simulink model "Integrate_velocity_to_position"  (R2018a)
settings: Solver=VariableStepAuto  StartTime=0.0  StopTime=10.0  RelTol=1e-3
values from neighbouring files (symbols this model uses):
  Rearth = 6371000    [setupandrun.m]
  thetaInit_BN = thetaInit_BN_deg * deg2rad    [setupandrun.m]
  xDotInit_E_B_BE = [150; 0; 0]    [setupandrun.m]
  xInit_E_E_BE = [Rearth; 0; 0]    [setupandrun.m]
settings Model: Creator=lamy  LastModifiedBy=lamy

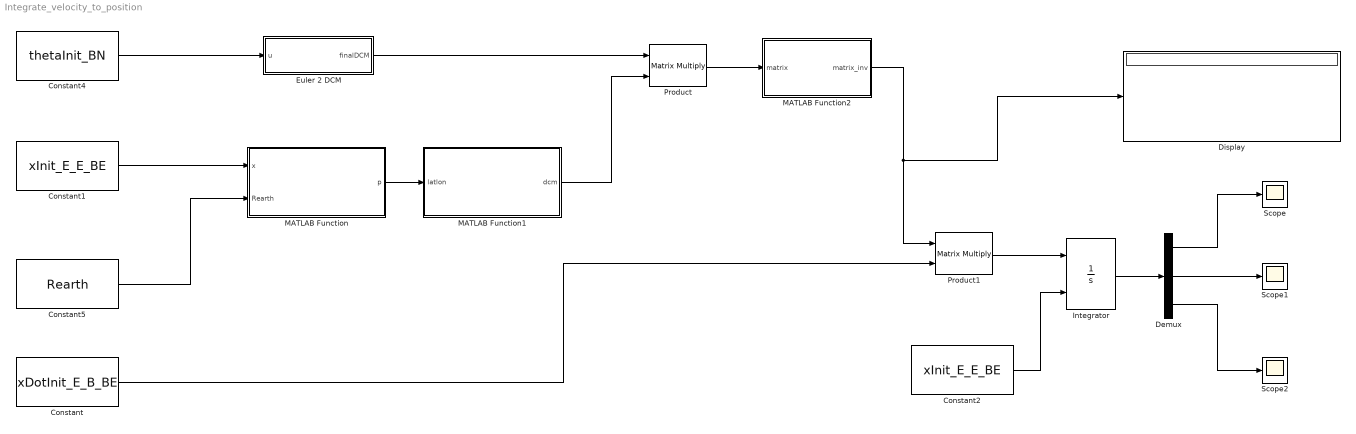
== system Integrate_velocity_to_position ==
  Constant : Constant  Value=xDotInit_E_B_BE
  Constant1 : Constant  Value=xInit_E_E_BE
  Constant2 : Constant  Value=xInit_E_E_BE
  Constant4 : Constant  Value=thetaInit_BN
  Constant5 : Constant  Value=Rearth
  Demux : Demux  Outputs=3
  Display : Display
  Euler 2 DCM : MATLAB Function  TreatAsAtomicUnit=on
  Integrator : Integrator  InitialConditionSource=external
  MATLAB Function : MATLAB Function  TreatAsAtomicUnit=on
  MATLAB Function1 : MATLAB Function  TreatAsAtomicUnit=on
  MATLAB Function2 : MATLAB Function  TreatAsAtomicUnit=on
  Product : Product  Multiplication=Matrix(*)
  Product1 : Product  Multiplication=Matrix(*)
  Scope : Scope
  Scope1 : Scope
  Scope2 : Scope
  wires:
  Constant4/1 -> Euler 2 DCM/1(u)
  Euler 2 DCM/1(finalDCM) -> Product/1
  Constant1/1 -> MATLAB Function/1(x)
  Constant5/1 -> MATLAB Function/2(Rearth)
  MATLAB Function/1(p) -> MATLAB Function1/1(latlon)
  MATLAB Function1/1(dcm) -> Product/2
  Product/1 -> MATLAB Function2/1(matrix)
  MATLAB Function2/1(matrix_inv) -> Display/1, Product1/1
  Constant/1 -> Product1/2
  Product1/1 -> Integrator/1
  Constant2/1 -> Integrator/2
  Integrator/1 -> Demux/1
  Demux/1 -> Scope/1
  Demux/2 -> Scope1/1
  Demux/3 -> Scope2/1

== matlab function Integrate_velocity_to_position/Euler 2 DCM ==
  data: u input; finalDCM output
function finalDCM = att2dcm(u)
yawDCM = [ cos(u(3)) sin(u(3)) 0 ;
-sin(u(3)) cos(u(3)) 0 ;
0 0 1 ];
pitchDCM = [ cos(u(2)) 0 -sin(u(2));
0 1 0 ;
sin(u(2)) 0 cos(u(2)) ];
rollDCM = [ 1 0 0 ;
0 cos(u(1)) sin(u(1));
0 -sin(u(1)) cos(u(1)) ];
finalDCM = rollDCM * pitchDCM * yawDCM;

== matlab function Integrate_velocity_to_position/MATLAB Function ==
  data: x input; p output; Rearth input
function p = cart2latlon(x,Rearth)
lat = atan2(x(3),sqrt(x(1)^2+x(2)^2));
lon = atan2(x(2),x(1));
alt = sqrt(x(1)^2+x(2)^2+x(3)^2) - Rearth;
p = [lat,lon,alt];

== matlab function Integrate_velocity_to_position/MATLAB Function1 ==
  data: latlon input; dcm output
function dcm = latlon2dcm(latlon)
dcm_lat = [cos(latlon(1)) 0 sin(latlon(1));
        0 1 0;
        -sin(latlon(1)) 0 cos(latlon(1))];
dcm_lon = [1 0 0;
    0 cos(latlon(2)) sin(latlon(2));
    0 -sin(latlon(2)) cos(latlon(2))];
constant = [0 0 1; 0 1 0;-1 0 0];
dcm = dcm_lat*dcm_lon*constant;

== matlab function Integrate_velocity_to_position/MATLAB Function2 ==
  data: matrix input; matrix_inv output
function matrix_inv = inverse(matrix)
matrix_inv = inv(matrix);
